simulink model "simCarro"  (R2022b)
settings: Solver=VariableStepAuto  StartTime=0.0  StopTime=Tsim  RelTol=1e-3
InitFcn:
  | fismovil = readfis("fismovil3.fis");
values from neighbouring files (symbols this model uses):
  fismovil3 = readfis("fismovil3.fis")    [init_Carro.m]
  piI = 0.5*pi    (= 1.57079632679)    [init_Carro.m]
  xf = 75    [init_Carro.m]
  xi = 10    [init_Carro.m]
  yf = 75    [init_Carro.m]
  yi = 10    [init_Carro.m]
libraries: fuzblock x1
settings Model: Creator=gadia  LastModifiedBy=gadia

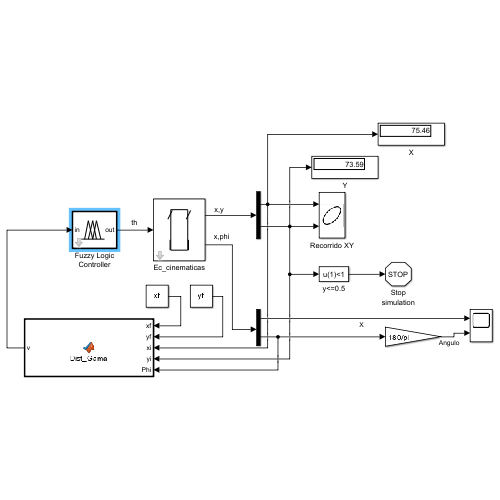
[thumbnail: Simulink's stored preview of the top-level diagram]
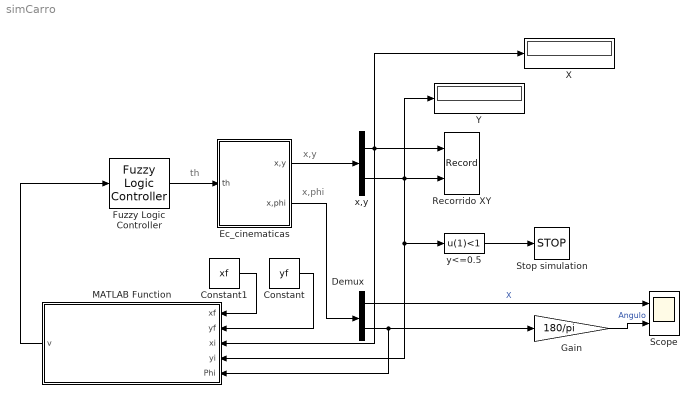
== system simCarro ==
  note: x,y
  note: x,phi
  note: th
  Constant : Constant  Value=yf
  Constant1 : Constant  Value=xf
  Demux : Demux  Outputs=2
  Ec_cinematicas : Subsystem  mask{X=xi, Y=yi, Phi=piI, D=2}
      mask prompts: X "Posición inicial X (0-100 cm):"; Y "Posición inical Y (0-100 cm):"; Phi "Orientación inicial Phi (-pi/2 a 3pi/2):"; D "Desplazamiento"
      mask Display: plot(-3, -3, 3, 3,[-1 1 1 -1 -1],[-2 -2 2 2 -2],[-1.1 -1.1],[-2 -1],[1.1 1.1],[-2 -1],[1.35 0.85],[1.93 1.07],[-0.85 -1.35],[1.93 1.07])
  Fuzzy Logic Controller : fuzblock/Fuzzy Logic  Controller  FIS=fismovil3  OutputSampleNumber=100  DataType=double  FuzzifiedInputs=off  RuleFiringStrengths=off  RuleOutputs=off  AggregatedOutputs=off  SimulateUsing=Interpreted execution  OutOfRangeInputValueMessage=warning  NoRuleFiredMessage=warning  EmptyOutputFuzzySetMessage=warning
  Gain : Gain  Gain=180/pi
  MATLAB Function : MATLAB Function  TreatAsAtomicUnit=on
  Recorrido XY : Record  FileSettingsInternal="{\"entries\":[{\"content\":{\"excelSettings\":{\"content\":{},\"type\":\"Streamout.ExcelSettings\"}},\"type\":\"Streamout.FileSettingStorage\",\"uuid\":\"\"}],\"packageUris\":[\"http:\\/\\/schema.mathworks.com\\/mf0\\/streamout_blocks\\/R2020a\"],\"version\":\"1.0\"}"  Layout=[1 1]  SignalsInternal="{\"entries\":[{\"content\":{\"signals\":[{\"content\":{\"blockPath\":[],\"channel\":[],\"dimensions\":[1],\"domain\":\"\",\"lineColor\":\"#77ac30\",\"plots\":[],\"port\":1,\"sid\":[\"\"],\"signalID\":438,\"signalName\":\"x,y:1\"},\"type\":\"RecordBlkView.Signal\",\"uuid\":\"\"},{\"content\":{\"blockPath\":[],\"channel\":[],\"dimensions\":[1],\"domain\":\"\",\"lineColor\":\"#4dbeee\",\"plots\":[],\"port\":2,\"sid\":[\"\"],\"signalID\":442,\"signalName\":\"x,y:2\"},\"type\":\"RecordBlkView.Signal\",\"uuid\":\"\"}]},\"type\":\"RecordBlkView.InputSignals\",\"uuid\":\"\"}],\"packageUris\":[\"http:\\/\\/schema.mathworks.com\\/mf0\\/streamout_blocks\\/R2020a\"],\"version\":\"1.0\"}"  VisualizationBindings="{\"xyplotplugin\":{\"info\":[{\"series\":[],\"subplotID\":1}]}}"  CompatibilityTag=XY  st=-1
  Scope : Scope  NumInputPorts=2
  Stop simulation : Stop
  X : Display
  Y : Display
  x,y : Demux  Outputs=2
  y<=0.5 : Fcn  Expr=u(1)<1
  wires:
  Gain/1 -> Scope/2  "Angulo"
  y<=0.5/1 -> Stop simulation/1
  Demux/1 -> Scope/1  "X"
  Fuzzy Logic Controller/1 -> Ec_cinematicas/1(th)
  Ec_cinematicas/1(x,y) -> x,y/1
  x,y/1 -> MATLAB Function/3(xi), X/1, Recorrido XY/1
  Ec_cinematicas/2(x,phi) -> Demux/1
  Demux/2 -> MATLAB Function/5(Phi), Gain/1
  x,y/2 -> Y/1, Recorrido XY/2, MATLAB Function/4(yi), y<=0.5/1
  MATLAB Function/1(v) -> Fuzzy Logic Controller/1
  Constant1/1 -> MATLAB Function/1(xf)
  Constant/1 -> MATLAB Function/2(yf)

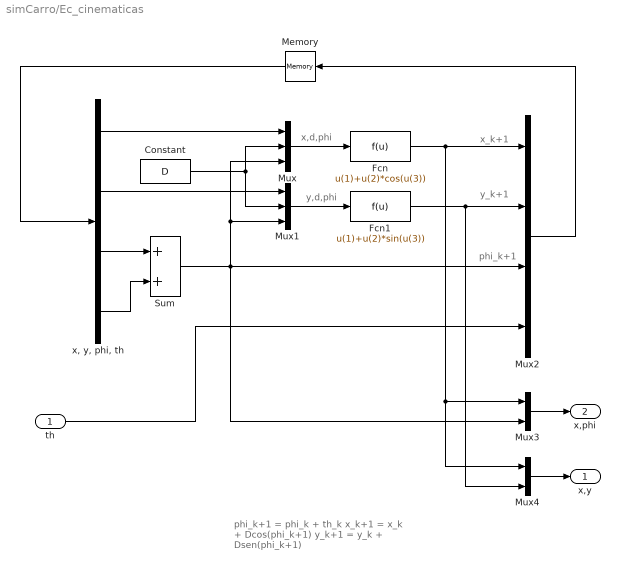
== system simCarro/Ec_cinematicas ==
  note: x,d,phi
  note: x_k+1
  note: y,d,phi
  note: y_k+1
  note: phi_k+1 = phi_k + th_k
      |
      | x_k+1 = x_k + Dcos(phi_k+1)
      |
      | y_k+1 = y_k + Dsen(phi_k+1)
  note: phi_k+1
  th : Inport
  Constant : Constant  Value=D
  Fcn : Fcn  Expr=u(1)+u(2)*cos(u(3))
  Fcn1 : Fcn  Expr=u(1)+u(2)*sin(u(3))
  Memory : Memory  InitialCondition=[X Y Phi 0]
  Mux : Mux  Inputs=3
  Mux1 : Mux  Inputs=3
  Mux2 : Mux
  Mux3 : Mux  Inputs=2
  Mux4 : Mux  Inputs=2
  Sum : Sum
  "x, y, phi, th" : Demux
  x,y : Outport
  x,phi : Outport  Port=2
  wires:
  Mux/1 -> Fcn/1
  Mux1/1 -> Fcn1/1
  Fcn/1 -> Mux2/1, Mux3/1, Mux4/1
  Fcn1/1 -> Mux2/2, Mux4/2
  "x, y, phi, th"/1 -> Mux/1
  "x, y, phi, th"/2 -> Mux1/1
  "x, y, phi, th"/3 -> Sum/1
  Sum/1 -> Mux1/3, Mux/3, Mux3/2, Mux2/3
  Constant/1 -> Mux/2, Mux1/2
  Mux3/1 -> x,phi/1
  Mux4/1 -> x,y/1
  th/1 -> Mux2/4
  "x, y, phi, th"/4 -> Sum/2
  Memory/1 -> "x, y, phi, th"/1
  Mux2/1 -> Memory/1

== matlab function simCarro/MATLAB Function ==
  data: xf input; v output; yf input; xi input; yi input; Phi input
%  Cálculo de la DISTANCIA  que separa al móvil de su
%  punto final y del ángulo GAMA necesario para calcular
%  el ángulo ALFA, perteneciente al sistema de conducción de un móvil
% u = [ xf ; yf ; xi ; yi ; Phi]
% v = [ Alfa ; Distancia ] 


function v = Dist_Gama(xf, yf, xi, yi, Phi)

% Cálculo de la distancia
  dX        = abs(xf - xi);
  dY        = abs(yf - yi); 
  distancia = sqrt(dX^2 + dY^2);
  cateto_opuesto = 0;
  Angulo_cuadrante = 0;
% Cálculo del cuadrante de operacion
  if (yf >= yi && xf > xi)
      Angulo_cuadrante = 0 ;
      cateto_opuesto   = dY ;
  end
  if (yf >= yi && xf <= xi)
      Angulo_cuadrante = pi/2 ;
      cateto_opuesto   = dX ;
  end
  if (yf < yi  && xf <= xi)
      Angulo_cuadrante = pi ;
      cateto_opuesto   = dY ;
  end
  if (yf < yi  && xf > xi)
      Angulo_cuadrante = 3*pi/2 ;
      cateto_opuesto   = dX ;
  end

% Cálculo del ángulo beta
  Beta      = asin(cateto_opuesto/distancia);
  
% Cálculo del ángulo gama
  Gama      = Beta + Angulo_cuadrante;

% Cálculo de Alfa conservando el rango entre -180 0 180
  Alfa      = Phi - Gama; 
  if  (Alfa > pi)
      Alfa  = Alfa - 2*pi;
  end
  if (Alfa < -pi)
      Alfa  = 2*pi + Alfa;
  end

  v = [Alfa;distancia];
end
